simulink model "RET_lab_4_Das_Sourav"  (R2016a)
settings: Solver=VariableStepAuto  StartTime=0.0  StopTime=0.5  RelTol=1e-3
libraries: powerlib x13, re_lib x2, simulink x1
settings Model: Creator=USER  LastModifiedBy=SD

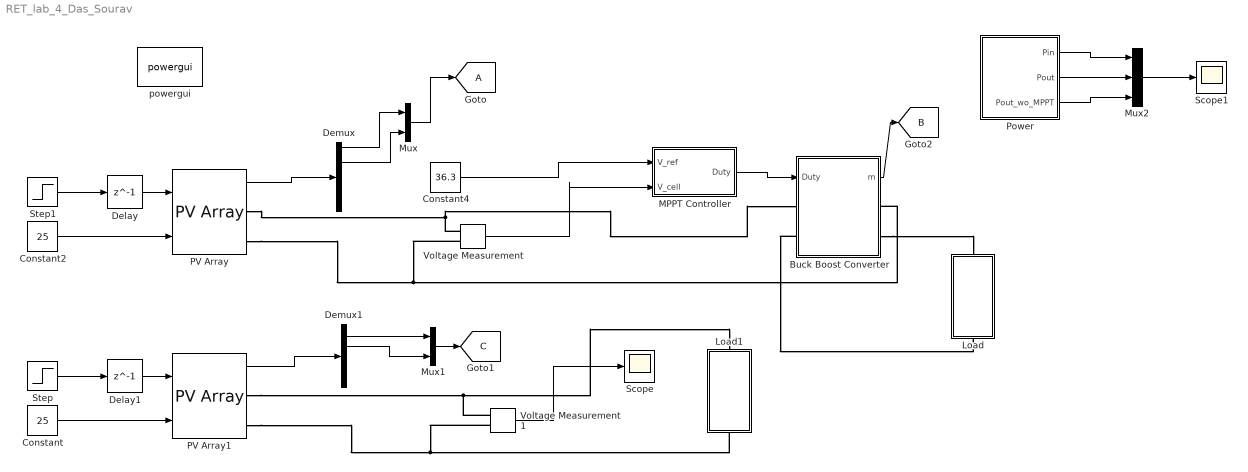
== system RET_lab_4_Das_Sourav ==
  Buck Boost Converter : Subsystem
  Constant : Constant  Value=25
  Constant2 : Constant  Value=25
  Constant4 : Constant  Value=36.3
  Delay : Delay  DelayLength=1  InitialCondition=0
  Delay1 : Delay  DelayLength=1  InitialCondition=0
  Demux : Demux  Outputs=5
  Demux1 : Demux  Outputs=5
  Load : Subsystem
  Load1 : Subsystem
  MPPT Controller : Subsystem
  Mux : Mux  Inputs=2
  Mux1 : Mux  Inputs=2
  Mux2 : Mux  Inputs=3
  PV Array : re_lib/Solar/PV Array  Npar=1  Nser=2  PlotType=array @ 1000 W/m2 & specified temperatures  S_vec="[ 1000  500  100 ]"  Temp_C_vec="[ 45 25  ]"  ModuleName=1Soltech 1STH-215-P  PlotWhenSelected=off  Pm=213.15  Ncell=60  Voc=36.3  Isc=7.84  Vm=29  Im=7.35  beta_Voc_pc=-0.36099  alpha_Isc_pc=0.102  beta_Voc=-0.13104  alpha_Isc=0.007997  IL=7.8649  I0=2.9259e-10  nI=0.98117  Rsh=313.3991  Rs=0.39383  BAL=off  Tc=1e-6  Tfilter=5e-5
  PV Array1 : re_lib/Solar/PV Array  Npar=1  Nser=2  PlotType=array @ 1000 W/m2 & specified temperatures  S_vec="[ 1000  500  100 ]"  Temp_C_vec="[ 45 25  ]"  ModuleName=1Soltech 1STH-215-P  PlotWhenSelected=off  Pm=213.15  Ncell=60  Voc=36.3  Isc=7.84  Vm=29  Im=7.35  beta_Voc_pc=-0.36099  alpha_Isc_pc=0.102  beta_Voc=-0.13104  alpha_Isc=0.007997  IL=7.8649  I0=2.9259e-10  nI=0.98117  Rsh=313.3991  Rs=0.39383  BAL=off  Tc=1e-6  Tfilter=5e-5
  Power : Subsystem
  Scope : Scope
  Scope1 : Scope
  Step : Step  Time=0  After=1000  SampleTime=1e-6
  Step1 : Step  Time=0  After=1000  SampleTime=1e-6
  Voltage Measurement : powerlib/Measurements/Voltage Measurement  PhasorSimulation=off  OutputType=Complex  PSBequivalent=0
  Voltage Measurement1 : powerlib/Measurements/Voltage Measurement  PhasorSimulation=off  OutputType=Complex  PSBequivalent=0
  powergui : powerlib/powergui  Priority=1  SimulationMode=Discrete  SolverType=Tustin/Backward Euler (TBE)  SampleTime=1e-06  frequency=60  SPID=off  DisableSnubberDevices=off  DisableRonSwitches=off  DisableVfSwitches=off  SwTol=0  DisplayEquations=off  Interpol=off  ExternalGateDelay=off  methode=off  Ts=10  FunctionMessages=off  echomessages=off  HookPort=off  EnableUseOfTLC=off  x0status=blocks  frequencyindice=0  Pbase=100e6  ErrMax=1e-4  Iterations=50  UnitsV=kV  UnitsW=MW  buscounter=0  RestoreLinks=warning  ResistiveCurrentMeasurement=off  Frange=[0:2:500]  Ylog=off  Xlog=on  ShowGrid=off  save=off  variable=ZData  structure=0  ZoomFFT=off  StartTime=0.0  cycles=1  DisplayStyle=1  fundamental=60  FreqAxis=off  MaxFrequency=1000  frequencyindicesteady=1  RmsSteady=1  display=off
  tag scope: A=global, B=global, C=global
  wires:
  PV Array/1 -> Demux/1
  Mux/1 -> [A]
  Voltage Measurement/1 -> MPPT Controller/2(V_cell)
  Constant4/1 -> MPPT Controller/1(V_ref)
  Constant2/1 -> PV Array/2
  MPPT Controller/1(Duty) -> Buck Boost Converter/1(Duty)
  Buck Boost Converter/1(m) -> [B]
  PV Array1/1 -> Demux1/1
  Demux1/1 -> Mux1/1
  Demux1/2 -> Mux1/2
  Mux1/1 -> [C]
  Voltage Measurement1/1 -> Scope/1
  Power/1(Pin) -> Mux2/1
  Power/2(Pout) -> Mux2/2
  Power/3(Pout_wo_MPPT) -> Mux2/3
  Mux2/1 -> Scope1/1
  Constant/1 -> PV Array1/2
  Step1/1 -> Delay/1
  Delay/1 -> PV Array/1
  Step/1 -> Delay1/1
  Delay1/1 -> PV Array1/1
  Demux/1 -> Mux/1
  Demux/2 -> Mux/2
  connections:
  PV Array/RConn1 -- Buck Boost Converter/LConn1 -- Voltage Measurement/LConn1
  PV Array/RConn2 -- Buck Boost Converter/RConn1 -- Voltage Measurement/LConn2
  Buck Boost Converter/LConn2 -- Load/RConn1
  Buck Boost Converter/RConn2 -- Load/LConn1
  PV Array1/RConn1 -- Voltage Measurement1/LConn1 -- Load1/RConn1
  PV Array1/RConn2 -- Voltage Measurement1/LConn2 -- Load1/LConn1

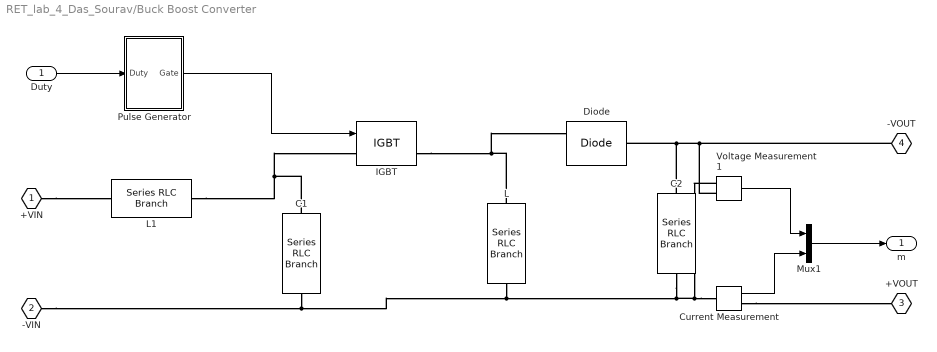
== system RET_lab_4_Das_Sourav/Buck Boost Converter ==
  Duty : Inport
  C1 : powerlib/Elements/Series RLC Branch  LConnTagsString=__new0  RConnTagsString=__new0  BranchType=C  Resistance=1  Inductance=1e-3  SetiL0=off  InitialCurrent=0  Capacitance=2000e-6  Setx0=off  InitialVoltage=0  Measurements=None
  C2 : powerlib/Elements/Series RLC Branch  LConnTagsString=__new0  RConnTagsString=__new0  BranchType=C  Resistance=1  Inductance=1e-3  SetiL0=off  InitialCurrent=0  Capacitance=2000e-6  Setx0=off  InitialVoltage=0  Measurements=None
  Current Measurement : powerlib/Measurements/Current Measurement  PhasorSimulation=off  OutputType=Complex  PSBequivalent=0
  Diode : powerlib/Power Electronics/Diode  Ron=0.001  Lon=0  Vf=0.8  IC=0  UseSnubber=off  Rs=500  Cs=250e-9  Measurements=on
  IGBT : powerlib/Power Electronics/IGBT  Ron=0.001  Lon=0  Vf=1  Tf=1e-6  Tt=2e-6  IC=0  Rs=1e5  Cs=inf  Measurements=on
  L : powerlib/Elements/Series RLC Branch  LConnTagsString=__new0  RConnTagsString=__new0  BranchType=L  Resistance=1  Inductance=47e-6  SetiL0=off  InitialCurrent=0  Capacitance=1e-6  Setx0=off  InitialVoltage=0  Measurements=None
  L1 : powerlib/Elements/Series RLC Branch  LConnTagsString=__new0  RConnTagsString=__new0  BranchType=L  Resistance=1000e-6  Inductance=1000e-6  SetiL0=off  InitialCurrent=0  Capacitance=1e-6  Setx0=off  InitialVoltage=0  Measurements=None
  Mux1 : Mux  Inputs=2
  Pulse Generator : Subsystem
  Voltage Measurement1 : powerlib/Measurements/Voltage Measurement  PhasorSimulation=off  OutputType=Complex  PSBequivalent=0
  +VIN : PMIOPort  Port=1  Side=Left
  -VIN : PMIOPort  Port=2  Side=Right
  +VOUT : PMIOPort  Port=3  Side=Left
  -VOUT : PMIOPort  Port=4  Side=Right
  m : Outport
  wires:
  Voltage Measurement1/1 -> Mux1/1
  Pulse Generator/1(Gate) -> IGBT/1
  Current Measurement/1 -> Mux1/2
  Mux1/1 -> m/1
  Duty/1 -> Pulse Generator/1(Duty)
  connections:
  Diode/LConn1 -- -VOUT/RConn1 -- Voltage Measurement1/LConn2 -- C2/LConn1
  L1/RConn1 -- C1/LConn1 -- IGBT/LConn1
  Current Measurement/RConn1 -- +VOUT/RConn1
  IGBT/RConn1 -- L/LConn1 -- Diode/RConn1
  Current Measurement/LConn1 -- -VIN/RConn1 -- C1/RConn1 -- L/RConn1 -- C2/RConn1 -- Voltage Measurement1/LConn1
  +VIN/RConn1 -- L1/LConn1

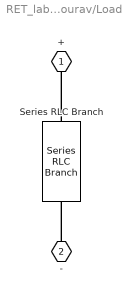
== system RET_lab_4_Das_Sourav/Load ==
  Series RLC Branch : powerlib/Elements/Series RLC Branch  LConnTagsString=__new0  RConnTagsString=__new0  BranchType=R  Resistance=60  Inductance=1e-3  SetiL0=off  InitialCurrent=0  Capacitance=1e-6  Setx0=off  InitialVoltage=0  Measurements=None
  + : PMIOPort  Port=1  Side=Right
  - : PMIOPort  Port=2  Side=Left
  connections:
  -/RConn1 -- Series RLC Branch/RConn1
  Series RLC Branch/LConn1 -- +/RConn1

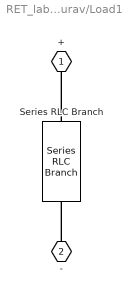
== system RET_lab_4_Das_Sourav/Load1 ==
  Series RLC Branch : powerlib/Elements/Series RLC Branch  LConnTagsString=__new0  RConnTagsString=__new0  BranchType=R  Resistance=60  Inductance=1e-3  SetiL0=off  InitialCurrent=0  Capacitance=1e-6  Setx0=off  InitialVoltage=0  Measurements=None
  + : PMIOPort  Port=1  Side=Right
  - : PMIOPort  Port=2  Side=Left
  connections:
  -/RConn1 -- Series RLC Branch/RConn1
  Series RLC Branch/LConn1 -- +/RConn1

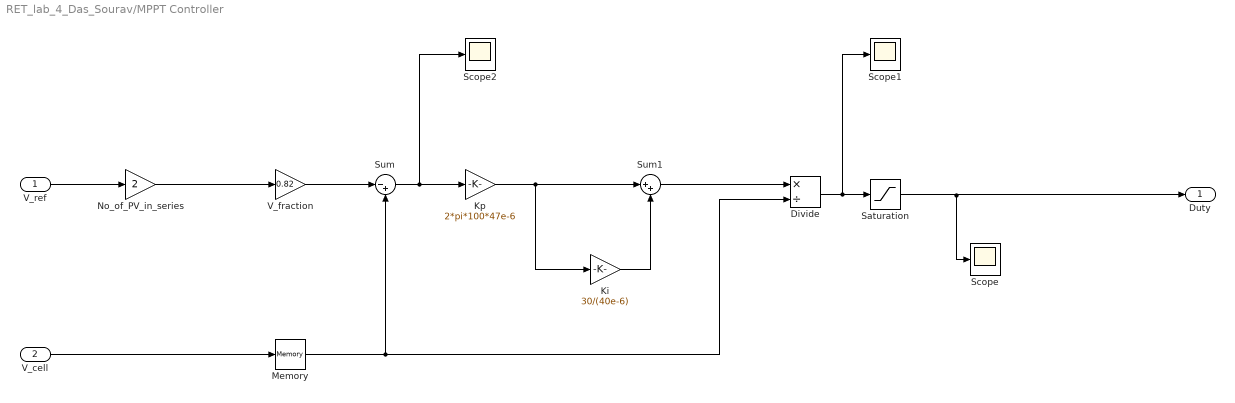
== system RET_lab_4_Das_Sourav/MPPT Controller ==
  V_ref : Inport
  V_cell : Inport  Port=2
  Divide : Product  Inputs=*/
  Ki : Gain  Gain=30/(40e-6)
  Kp : Gain  Gain=2*pi*100*47e-6
  Memory : Memory
  No_of_PV_in_series : Gain  Gain=2
  Saturation : Saturate
  Scope : Scope
  Scope1 : Scope
  Scope2 : Scope
  Sum : Sum  Inputs=|-+
  Sum1 : Sum  Inputs=|++
  "V_fraction " : Gain  Gain=0.82
  Duty : Outport
  wires:
  V_ref/1 -> No_of_PV_in_series/1
  Memory/1 -> Divide/2, Sum/2
  Kp/1 -> Ki/1, Sum1/1
  Saturation/1 -> Duty/1, Scope/1
  No_of_PV_in_series/1 -> "V_fraction "/1
  "V_fraction "/1 -> Sum/1
  V_cell/1 -> Memory/1
  Sum/1 -> Scope2/1, Kp/1
  Divide/1 -> Scope1/1, Saturation/1
  Sum1/1 -> Divide/1
  Ki/1 -> Sum1/2

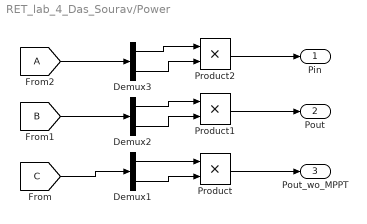
== system RET_lab_4_Das_Sourav/Power ==
  Demux1 : Demux  Outputs=2
  Demux2 : Demux  Outputs=2
  Demux3 : Demux  Outputs=2
  Product : Product
  Product1 : Product
  Product2 : Product
  Pin : Outport
  Pout : Outport  Port=2
  Pout_wo_MPPT : Outport  Port=3
  wires:
  Demux3/1 -> Product2/1
  Demux2/1 -> Product1/1
  [C] -> Demux1/1
  [A] -> Demux3/1
  Demux1/2 -> Product/2
  Demux3/2 -> Product2/2
  Demux1/1 -> Product/1
  Demux2/2 -> Product1/2
  Product2/1 -> Pin/1
  Product1/1 -> Pout/1
  [B] -> Demux2/1
  Product/1 -> Pout_wo_MPPT/1

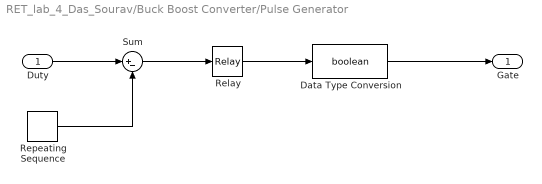
== system RET_lab_4_Das_Sourav/Buck Boost Converter/Pulse Generator ==
  Duty : Inport
  Data Type Conversion : DataTypeConversion  OutDataTypeStr=boolean  RndMeth=Zero
  Relay : Relay
  Repeating Sequence : simulink/Sources/Repeating Sequence  rep_seq_t=[0 1/10e3]  rep_seq_y=[0 1]
  Sum : Sum  Inputs=|+-
  Gate : Outport
  wires:
  Sum/1 -> Relay/1
  Data Type Conversion/1 -> Gate/1
  Duty/1 -> Sum/1
  Relay/1 -> Data Type Conversion/1
  Repeating Sequence/1 -> Sum/2
